simulink model "pfa1008"  (R2025a)
settings: Solver=VariableStepAuto  StartTime=0.0  StopTime=1e-4  RelTol=1e-3
InitFcn:
  | coeffs;
undefined symbols (not defined in the file or in its folder): S, vsva2197, xcvc1902
libraries: aieBasic x20, aieUtilities x5, dspsrcs4 x4, hlsBasic x2, vmcUtilities x1
(part 2 of 2)

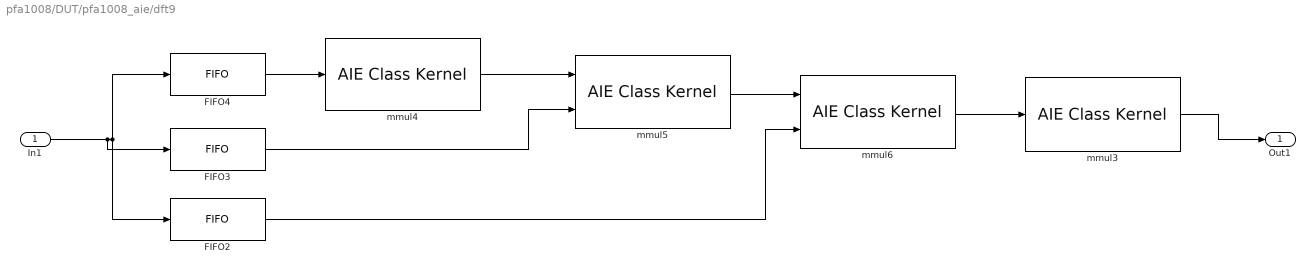
== system pfa1008/DUT/pfa1008_aie/dft9 ==
  In1 : Inport
  FIFO2 : aieBasic/FIFO  FifoDepth=32  FIFOType=0  TileType=0  RowLocation=0  ColLocation=0  channel=0  blockJsonConstraints=[]  deprecateConstraints=0
  FIFO3 : aieBasic/FIFO  FifoDepth=32  FIFOType=0  TileType=0  RowLocation=0  ColLocation=0  channel=0  blockJsonConstraints=[]  deprecateConstraints=0
  FIFO4 : aieBasic/FIFO  FifoDepth=32  FIFOType=0  TileType=0  RowLocation=0  ColLocation=0  channel=0  blockJsonConstraints=[]  deprecateConstraints=0
  mmul3 : aieBasic/AIE Class Kernel  KernelAllAttrs=|  PortNames={'acc_i'; 'sig_o'}  PortSerializedTypes={'{Q2{P{Tinput_cascade{2{t{Scacc64}}{t{Bv}}}}}}'; '{Q2{R{Tadf::output_buffer{2{t{Scint16}}{t{Tadf::extents{1{t{}1008}}}}}}}}'}  PortWindowSizes={0.000000000000000000e+00; 1.008000000000000000e+03}  PortWindowMargins={0.000000000000000000e+00; 0.000000000000000000e+00}  PortSynchronicities={'auto', 'sync'}  PortSignalSizes={0.000000000000000000e+00; 0.000000000000000000e+00}  ClassTemplateSpecKind=none  ClassTemplateParamNames={}  ClassTemplateParamKinds={}  ClassTemplateParamTypes={}  ClassTemplateParamValues={}  ClassCtorParamNames={}  ClassCtorParamSerializedTypes={}  ClassCtorParamValues={}  ClassIndex=1  ClassCtorIndex=0  ClassTabVisible=on  ClassTemplateParamsVisible=off  ClassCtorDeclVisible=off  ClassCtorParamsVisible=off  FunctionTabVisible=on  FunctionDecl=|  PortAttrs={ 'input', 'acc_i', 'input_cascade< cacc64, void > * restrict', '', '', '', ''; 'output', 'sig_o', 'adf::output_buffer< cint16, adf::extents< 1008 > > & restrict', '1008', '', 'sync', '' }  PortAttrsEnables={'off', 'off', 'off', 'off', 'off', 'off', 'off';'off', 'off', 'off', 'off', 'off', 'off', 'off'}  SampleTime=-1  ClassDeclTypeOptions=C[1 1]@t13@class dft9_3;  ClassDecl=class dft9_3;  ClassTemplateParams={}  ClassTemplateParamsEnables={}  ClassCtorDeclTypeOptions=C[1 1]@t7@<empty>  ClassCtorDecl=<empty>  ClassCtorParams={}  KernelHeaderFile=dft9_mmul3.h  KernelClassName=dft9_3  KernelFunction=run  KernelSourceFile=dft9_mmul3.cpp  KernelSearchPaths={'./aie/dft9'}  PreProcOptions={}  blockJsonConstraints=[]
      KernelAllAttrs=|
      | s[12;12;9;9;19;14;21;23;21;23;24;21;15;17;12;24;26;26;26;27;28;9;21;23;23;23;24;25;14;19;19;29]@FunctionNameDeclFileNamePortNamesPortTypesPortSerializedTypesPortDirectionsPortWindowSizeEnablesPortWindowMarginEnablesPortBufferSizeEnablesPortBufferMarginEnablesPortSynchronicityEnablesPortSignalSizeEnablesPortBufferSizesPortBufferMarginsFunctionDeclFunctionTemplateSpecKindFunctionTemplateParamNamesFunctionTemplateParamKindsFunctionTemplateParamTypesFunctionTemplateParamValuesFunctionTemplateParamEnablesClassDeclClassTemplateSpecKindClassTemplateParamNamesClassTemplateParamKindsClassTemplateParamTypesClassTemplateParamValuesClassTemplateParamEnablesClassCtorDeclsClassCtorParamNamesClassCtorParamTypesClassCtorParamSerializedTypes[1 1]@C[32 1]@t3@runt26@../../../dft9/dft9_mmul3.hC[2 1]@t5@acc_it5@sig_oC[2 1]@t40@input_cascade< cacc64, void > * restrictt61@adf::output_buffer< cint16, adf::extents< 1008 > > & restrictC[2 1]@t45@{Q2{P{Tinput_cascade{2{t{Scacc64}}{t{Bv}}}}}}t73@{Q2{R{Tadf::output_buffer{2{t{Scint16}}{t{Tadf::extents{1{t{}1008}}}}}}}}C[2 1]@t5@inputt6@outputC[2 1]@l0@l1@C[2 1]@l0@l0@C[2 1]@l0@l1@C[2 1]@l0@l0@C[2 1]@l0@l1@C[2 1]@l0@l0@C[2 1]@nt4@1008C[2 1]@nnt134@void dft9_3::
      | run(input_cascade< cacc64, void > * restrict acc_i, adf::output_buffer< cint16, adf::extents< 1008 > > & restrict sig_o)t4@nonee[0 1]@e[0 1]@e[0 1]@e[0 1]@e[0 1]@t13@class dft9_3;t4@nonee[0 1]@e[0 1]@e[0 1]@e[0 1]@e[0 1]@e[0 1]@e[0 1]@e[0 1]@e[0 1]@
      FunctionDecl=|
      | void dft9_3::
      | run(input_cascade< cacc64, void > * restrict acc_i, adf::output_buffer< cint16, adf::extents< 1008 > > & restrict sig_o)
  mmul4 : aieBasic/AIE Class Kernel  KernelAllAttrs=|  PortNames={'sig_i'; 'acc_o'}  PortSerializedTypes={'{Q2{R{Tadf::input_buffer{2{t{Scint16}}{t{Tadf::extents{1{t{}1008}}}}}}}}'; '{Q2{P{Toutput_cascade{2{t{Scacc64}}{t{Bv}}}}}}'}  PortWindowSizes={1.008000000000000000e+03; 0.000000000000000000e+00}  PortWindowMargins={0.000000000000000000e+00; 0.000000000000000000e+00}  PortSynchronicities={'sync', 'auto'}  PortSignalSizes={0.000000000000000000e+00; 2.016000000000000000e+03}  ClassTemplateSpecKind=none  ClassTemplateParamNames={}  ClassTemplateParamKinds={}  ClassTemplateParamTypes={}  ClassTemplateParamValues={}  ClassCtorParamNames={'coeff_i'}  ClassCtorParamSerializedTypes={'{R{C{Scint16}64}}'}  ClassCtorParamValues={'[32767;32767;32767;32767;32767;32767;32767;32767;32767;25102-21063i;5690-32270i;-16384-28378i;-30792-11207i;-30792+11207i;-16384+28378i;5690+32270i;32767;5690-32270i;-30792-11207i;-16384+28378i;25102+21063i;25102-21063i;-16384-28378i;-30792+11207i;32767;-16384-28378i;-16384+28378i;32767;-16384-28378i;-16384+28378i;32767;-16384-28378i;32767;0;0;0;0;0;0;0;25102+21063i;0;0;0;0;0;0;0;5690+32270i;0;0;0;0;0;0;0;-16384+28378i;0;0;0;0;0;0;0]'}  ClassIndex=1  ClassCtorIndex=1  ClassTabVisible=on  ClassTemplateParamsVisible=off  ClassCtorDeclVisible=on  ClassCtorParamsVisible=on  FunctionTabVisible=on  FunctionDecl=|  PortAttrs={ 'input', 'sig_i', 'adf::input_buffer< cint16, adf::extents< 1008 > > & restrict', '1008', '0', 'sync', ''; 'output', 'acc_o', 'output_cascade< cacc64, void > * restrict', '', '', '', '2016' }  PortAttrsEnables={'off', 'off', 'off', 'off', 'off', 'off', 'off';'off', 'off', 'off', 'off', 'off', 'off', 'on'}  SampleTime=-1  ClassDeclTypeOptions=C[1 1]@t13@class dft9_0;  ClassDecl=class dft9_0;  ClassTemplateParams={}  ClassTemplateParamsEnables={}  ClassCtorDeclTypeOptions=C[1 1]@t35@dft9_0(cint16 ( & coeff_i ) [ 64 ])  ClassCtorDecl=dft9_0(cint16 ( & coeff_i ) [ 64 ])  ClassCtorParams={ 'coeff_i', 'cint16 ( &) [ 64 ]', 'DFT9_TWID0' }  KernelHeaderFile=dft9_mmul0.h  KernelClassName=dft9_0  KernelFunction=run  KernelSourceFile=dft9_mmul0.cpp  KernelSearchPaths={'./aie/dft9'}  PreProcOptions={}  blockJsonConstraints=[]
      KernelAllAttrs=|
      | s[12;12;9;9;19;14;21;23;21;23;24;21;15;17;12;24;26;26;26;27;28;9;21;23;23;23;24;25;14;19;19;29]@FunctionNameDeclFileNamePortNamesPortTypesPortSerializedTypesPortDirectionsPortWindowSizeEnablesPortWindowMarginEnablesPortBufferSizeEnablesPortBufferMarginEnablesPortSynchronicityEnablesPortSignalSizeEnablesPortBufferSizesPortBufferMarginsFunctionDeclFunctionTemplateSpecKindFunctionTemplateParamNamesFunctionTemplateParamKindsFunctionTemplateParamTypesFunctionTemplateParamValuesFunctionTemplateParamEnablesClassDeclClassTemplateSpecKindClassTemplateParamNamesClassTemplateParamKindsClassTemplateParamTypesClassTemplateParamValuesClassTemplateParamEnablesClassCtorDeclsClassCtorParamNamesClassCtorParamTypesClassCtorParamSerializedTypes[1 1]@C[32 1]@t3@runt26@../../../dft9/dft9_mmul0.hC[2 1]@t5@sig_it5@acc_oC[2 1]@t60@adf::input_buffer< cint16, adf::extents< 1008 > > & restrictt41@output_cascade< cacc64, void > * restrictC[2 1]@t72@{Q2{R{Tadf::input_buffer{2{t{Scint16}}{t{Tadf::extents{1{t{}1008}}}}}}}}t46@{Q2{P{Toutput_cascade{2{t{Scacc64}}{t{Bv}}}}}}C[2 1]@t5@inputt6@outputC[2 1]@l1@l0@C[2 1]@l1@l0@C[2 1]@l1@l0@C[2 1]@l0@l0@C[2 1]@l1@l0@C[2 1]@l0@l1@C[2 1]@t4@1008nC[2 1]@nnt134@void dft9_0::
      | run(adf::input_buffer< cint16, adf::extents< 1008 > > & restrict sig_i, output_cascade< cacc64, void > * restrict acc_o)t4@nonee[0 1]@e[0 1]@e[0 1]@e[0 1]@e[0 1]@t13@class dft9_0;t4@nonee[0 1]@e[0 1]@e[0 1]@e[0 1]@e[0 1]@C[1 1]@t35@dft9_0(cint16 ( & coeff_i ) [ 64 ])C[1 1]@C[1 1]@t7@coeff_iC[1 1]@C[1 1]@t18@cint16 ( &) [ 64 ]C[1 1]@C[1 1]@t17@{R{C{Scint16}64}}
      FunctionDecl=|
      | void dft9_0::
      | run(adf::input_buffer< cint16, adf::extents< 1008 > > & restrict sig_i, output_cascade< cacc64, void > * restrict acc_o)
  mmul5 : aieBasic/AIE Class Kernel  KernelAllAttrs=|  PortNames={'acc_i'; 'sig_i'; 'acc_o'}  PortSerializedTypes={'{Q2{P{Tinput_cascade{2{t{Scacc64}}{t{Bv}}}}}}'; '{Q2{R{Tadf::input_buffer{2{t{Scint16}}{t{Tadf::extents{1{t{}1008}}}}}}}}'; '{Q2{P{Toutput_cascade{2{t{Scacc64}}{t{Bv}}}}}}'}  PortWindowSizes={0.000000000000000000e+00; 1.008000000000000000e+03; 0.000000000000000000e+00}  PortWindowMargins={0.000000000000000000e+00; 0.000000000000000000e+00; 0.000000000000000000e+00}  PortSynchronicities={'auto', 'sync', 'auto'}  PortSignalSizes={0.000000000000000000e+00; 0.000000000000000000e+00; 2.016000000000000000e+03}  ClassTemplateSpecKind=none  ClassTemplateParamNames={}  ClassTemplateParamKinds={}  ClassTemplateParamTypes={}  ClassTemplateParamValues={}  ClassCtorParamNames={'coeff_i'}  ClassCtorParamSerializedTypes={'{R{C{Scint16}64}}'}  ClassCtorParamValues={'[32767;-30792-11207i;25102+21063i;-16384-28378i;5690+32270i;5690-32270i;-16384+28378i;25102-21063i;32767;-30792+11207i;25102-21063i;-16384+28378i;5690-32270i;5690+32270i;-16384-28378i;25102+21063i;32767;-16384+28378i;-16384-28378i;32767;-16384+28378i;-16384-28378i;32767;-16384+28378i;32767;5690+32270i;-30792+11207i;-16384-28378i;25102-21063i;25102+21063i;-16384+28378i;-30792-11207i;-30792+11207i;0;0;0;0;0;0;0;-30792-11207i;0;0;0;0;0;0;0;-16384-28378i;0;0;0;0;0;0;0;5690-32270i;0;0;0;0;0;0;0]'}  ClassIndex=1  ClassCtorIndex=1  ClassTabVisible=on  ClassTemplateParamsVisible=off  ClassCtorDeclVisible=on  ClassCtorParamsVisible=on  FunctionTabVisible=on  FunctionDecl=|  PortAttrs={ 'input', 'acc_i', 'input_cascade< cacc64, void > * restrict', '', '', '', ''; 'input', 'sig_i', 'adf::input_buffer< cint16, adf::extents< 1008 > > & restrict', '1008', '0', 'sync', ''; 'output', 'acc_o', 'output_cascade< cacc64, void > * restrict', '', '', '', '2016' }  PortAttrsEnables={'off', 'off', 'off', 'off', 'off', 'off', 'off';'off', 'off', 'off', 'off', 'off', 'off', 'off';'off', 'off', 'off', 'off', 'off', 'off', 'on'}  SampleTime=-1  ClassDeclTypeOptions=C[1 1]@t13@class dft9_1;  ClassDecl=class dft9_1;  ClassTemplateParams={}  ClassTemplateParamsEnables={}  ClassCtorDeclTypeOptions=C[1 1]@t35@dft9_1(cint16 ( & coeff_i ) [ 64 ])  ClassCtorDecl=dft9_1(cint16 ( & coeff_i ) [ 64 ])  ClassCtorParams={ 'coeff_i', 'cint16 ( &) [ 64 ]', 'DFT9_TWID1' }  KernelHeaderFile=dft9_mmul1.h  KernelClassName=dft9_1  KernelFunction=run  KernelSourceFile=dft9_mmul1.cpp  KernelSearchPaths={'./aie/dft9'}  PreProcOptions={}  blockJsonConstraints=[]
      KernelAllAttrs=|
      | s[12;12;9;9;19;14;21;23;21;23;24;21;15;17;12;24;26;26;26;27;28;9;21;23;23;23;24;25;14;19;19;29]@FunctionNameDeclFileNamePortNamesPortTypesPortSerializedTypesPortDirectionsPortWindowSizeEnablesPortWindowMarginEnablesPortBufferSizeEnablesPortBufferMarginEnablesPortSynchronicityEnablesPortSignalSizeEnablesPortBufferSizesPortBufferMarginsFunctionDeclFunctionTemplateSpecKindFunctionTemplateParamNamesFunctionTemplateParamKindsFunctionTemplateParamTypesFunctionTemplateParamValuesFunctionTemplateParamEnablesClassDeclClassTemplateSpecKindClassTemplateParamNamesClassTemplateParamKindsClassTemplateParamTypesClassTemplateParamValuesClassTemplateParamEnablesClassCtorDeclsClassCtorParamNamesClassCtorParamTypesClassCtorParamSerializedTypes[1 1]@C[32 1]@t3@runt26@../../../dft9/dft9_mmul1.hC[3 1]@t5@acc_it5@sig_it5@acc_oC[3 1]@t40@input_cascade< cacc64, void > * restrictt60@adf::input_buffer< cint16, adf::extents< 1008 > > & restrictt41@output_cascade< cacc64, void > * restrictC[3 1]@t45@{Q2{P{Tinput_cascade{2{t{Scacc64}}{t{Bv}}}}}}t72@{Q2{R{Tadf::input_buffer{2{t{Scint16}}{t{Tadf::extents{1{t{}1008}}}}}}}}t46@{Q2{P{Toutput_cascade{2{t{Scacc64}}{t{Bv}}}}}}C[3 1]@t5@inputt5@inputt6@outputC[3 1]@l0@l1@l0@C[3 1]@l0@l1@l0@C[3 1]@l0@l1@l0@C[3 1]@l0@l0@l0@C[3 1]@l0@l1@l0@C[3 1]@l0@l0@l1@C[3 1]@nt4@1008nC[3 1]@nnnt182@void dft9_1::
      | run(input_cascade< cacc64, void > * restrict acc_i, adf::input_buffer< cint16, adf::extents< 1008 > > & restrict sig_i, output_cascade< cacc64, void > * restrict acc_o)t4@nonee[0 1]@e[0 1]@e[0 1]@e[0 1]@e[0 1]@t13@class dft9_1;t4@nonee[0 1]@e[0 1]@e[0 1]@e[0 1]@e[0 1]@C[1 1]@t35@dft9_1(cint16 ( & coeff_i ) [ 64 ])C[1 1]@C[1 1]@t7@coeff_iC[1 1]@C[1 1]@t18@cint16 ( &) [ 64 ]C[1 1]@C[1 1]@t17@{R{C{Scint16}64}}
      FunctionDecl=|
      | void dft9_1::
      | run(input_cascade< cacc64, void > * restrict acc_i, adf::input_buffer< cint16, adf::extents< 1008 > > & restrict sig_i, output_cascade< cacc64, void > * restrict acc_o)
  mmul6 : aieBasic/AIE Class Kernel  KernelAllAttrs=|  PortNames={'acc_i'; 'sig_i'; 'acc_o'}  PortSerializedTypes={'{Q2{P{Tinput_cascade{2{t{Scacc64}}{t{Bv}}}}}}'; '{Q2{R{Tadf::input_buffer{2{t{Scint16}}{t{Tadf::extents{1{t{}1008}}}}}}}}'; '{Q2{P{Toutput_cascade{2{t{Scacc64}}{t{Bv}}}}}}'}  PortWindowSizes={0.000000000000000000e+00; 1.008000000000000000e+03; 0.000000000000000000e+00}  PortWindowMargins={0.000000000000000000e+00; 0.000000000000000000e+00; 0.000000000000000000e+00}  PortSynchronicities={'auto', 'sync', 'auto'}  PortSignalSizes={0.000000000000000000e+00; 0.000000000000000000e+00; 2.016000000000000000e+03}  ClassTemplateSpecKind=none  ClassTemplateParamNames={}  ClassTemplateParamKinds={}  ClassTemplateParamTypes={}  ClassTemplateParamValues={}  ClassCtorParamNames={'coeff_i'}  ClassCtorParamSerializedTypes={'{R{C{Scint16}64}}'}  ClassCtorParamValues={'[32767;25102+21063i;5690+32270i;-16384+28378i;-30792+11207i;-30792-11207i;-16384-28378i;5690-32270i;0;0;0;0;0;0;0;0;0;0;0;0;0;0;0;0;0;0;0;0;0;0;0;0;25102-21063i;0;0;0;0;0;0;0;0;0;0;0;0;0;0;0;0;0;0;0;0;0;0;0;0;0;0;0;0;0;0;0]'}  ClassIndex=1  ClassCtorIndex=1  ClassTabVisible=on  ClassTemplateParamsVisible=off  ClassCtorDeclVisible=on  ClassCtorParamsVisible=on  FunctionTabVisible=on  FunctionDecl=|  PortAttrs={ 'input', 'acc_i', 'input_cascade< cacc64, void > * restrict', '', '', '', ''; 'input', 'sig_i', 'adf::input_buffer< cint16, adf::extents< 1008 > > & restrict', '1008', '0', 'sync', ''; 'output', 'acc_o', 'output_cascade< cacc64, void > * restrict', '', '', '', '2016' }  PortAttrsEnables={'off', 'off', 'off', 'off', 'off', 'off', 'off';'off', 'off', 'off', 'off', 'off', 'off', 'off';'off', 'off', 'off', 'off', 'off', 'off', 'on'}  SampleTime=-1  ClassDeclTypeOptions=C[1 1]@t13@class dft9_2;  ClassDecl=class dft9_2;  ClassTemplateParams={}  ClassTemplateParamsEnables={}  ClassCtorDeclTypeOptions=C[1 1]@t35@dft9_2(cint16 ( & coeff_i ) [ 64 ])  ClassCtorDecl=dft9_2(cint16 ( & coeff_i ) [ 64 ])  ClassCtorParams={ 'coeff_i', 'cint16 ( &) [ 64 ]', 'DFT9_TWID2' }  KernelHeaderFile=dft9_mmul2.h  KernelClassName=dft9_2  KernelFunction=run  KernelSourceFile=dft9_mmul2.cpp  KernelSearchPaths={'./aie/dft9'}  PreProcOptions={}  blockJsonConstraints=[]
      KernelAllAttrs=|
      | s[12;12;9;9;19;14;21;23;21;23;24;21;15;17;12;24;26;26;26;27;28;9;21;23;23;23;24;25;14;19;19;29]@FunctionNameDeclFileNamePortNamesPortTypesPortSerializedTypesPortDirectionsPortWindowSizeEnablesPortWindowMarginEnablesPortBufferSizeEnablesPortBufferMarginEnablesPortSynchronicityEnablesPortSignalSizeEnablesPortBufferSizesPortBufferMarginsFunctionDeclFunctionTemplateSpecKindFunctionTemplateParamNamesFunctionTemplateParamKindsFunctionTemplateParamTypesFunctionTemplateParamValuesFunctionTemplateParamEnablesClassDeclClassTemplateSpecKindClassTemplateParamNamesClassTemplateParamKindsClassTemplateParamTypesClassTemplateParamValuesClassTemplateParamEnablesClassCtorDeclsClassCtorParamNamesClassCtorParamTypesClassCtorParamSerializedTypes[1 1]@C[32 1]@t3@runt26@../../../dft9/dft9_mmul2.hC[3 1]@t5@acc_it5@sig_it5@acc_oC[3 1]@t40@input_cascade< cacc64, void > * restrictt60@adf::input_buffer< cint16, adf::extents< 1008 > > & restrictt41@output_cascade< cacc64, void > * restrictC[3 1]@t45@{Q2{P{Tinput_cascade{2{t{Scacc64}}{t{Bv}}}}}}t72@{Q2{R{Tadf::input_buffer{2{t{Scint16}}{t{Tadf::extents{1{t{}1008}}}}}}}}t46@{Q2{P{Toutput_cascade{2{t{Scacc64}}{t{Bv}}}}}}C[3 1]@t5@inputt5@inputt6@outputC[3 1]@l0@l1@l0@C[3 1]@l0@l1@l0@C[3 1]@l0@l1@l0@C[3 1]@l0@l0@l0@C[3 1]@l0@l1@l0@C[3 1]@l0@l0@l1@C[3 1]@nt4@1008nC[3 1]@nnnt182@void dft9_2::
      | run(input_cascade< cacc64, void > * restrict acc_i, adf::input_buffer< cint16, adf::extents< 1008 > > & restrict sig_i, output_cascade< cacc64, void > * restrict acc_o)t4@nonee[0 1]@e[0 1]@e[0 1]@e[0 1]@e[0 1]@t13@class dft9_2;t4@nonee[0 1]@e[0 1]@e[0 1]@e[0 1]@e[0 1]@C[1 1]@t35@dft9_2(cint16 ( & coeff_i ) [ 64 ])C[1 1]@C[1 1]@t7@coeff_iC[1 1]@C[1 1]@t18@cint16 ( &) [ 64 ]C[1 1]@C[1 1]@t17@{R{C{Scint16}64}}
      FunctionDecl=|
      | void dft9_2::
      | run(input_cascade< cacc64, void > * restrict acc_i, adf::input_buffer< cint16, adf::extents< 1008 > > & restrict sig_i, output_cascade< cacc64, void > * restrict acc_o)
  Out1 : Outport
  wires:
  FIFO2/1 -> mmul6/2
  mmul6/1 -> mmul3/1
  FIFO4/1 -> mmul4/1
  FIFO3/1 -> mmul5/2
  mmul4/1 -> mmul5/1
  mmul3/1 -> Out1/1
  mmul5/1 -> mmul6/1
  In1/1 -> FIFO2/1, FIFO4/1, FIFO3/1
